simulink model "s0809"  (Simulink 6.0)
settings: Solver=ode45  SolverMode=SingleTasking  StartTime=0.0  StopTime=300  MaxStep=200  RelTol=1e-3  AbsTol=1e-6
values from neighbouring files (symbols this model uses):
  T = 1    [m0304.m]
settings Model: LastModifiedBy=Froriep
settings DataIOCC: LimitDataPoints=off  SaveOutput=off  TimeSaveName=t
settings OptimizationCC: BooleanDataType=off
settings DebuggingCC: SolverPrmCheckMsg=none
settings HardwareCC: TargetUnknown=on
settings STFCustomTargetCC: TargetFcnLib=ansi_tfl_tmw.mat  GenFloatMathFcnCalls=ANSI_C  ModelReferenceCompliant=off  SystemTargetFile=grt.tlc

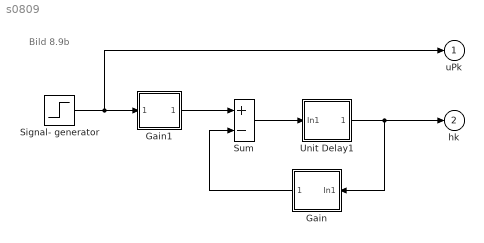
== system s0809 ==
  note: Bild 8.9b
  Gain : Subsystem  Orientation=left  mask{@1=a1}
      mask prompts: @1 "a1"
      mask help: Konstante
      mask init:
      | a1=@1;
      mask Display: disp('a1')
  Gain1 : Subsystem  mask{@1=b1}
      mask prompts: @1 "b0"
      mask help: Konstante
      mask init:
      | b1=@1;
      mask Display: disp('b1')
  Signal- generator : Step  Time=0  SampleTime=T
  Sum : Sum  Inputs=+-  SaturateOnIntegerOverflow=on  InputSameDT=on
  Unit Delay1 : Subsystem  mask{@1=T}
      mask prompts: @1 "T"
      mask help: Verschiebeglied
      mask init:
      | T=@1;
      mask Display: disp('T')
  uPk : Outport
  hk : Outport  Port=2
  wires:
  Signal- generator/1 -> uPk/1, Gain1/1(In1)
  Sum/1 -> Unit Delay1/1(In1)
  Gain1/1(Out1) -> Sum/1
  Gain/1(Out1) -> Sum/2
  Unit Delay1/1(Out1) -> Gain/1(In1), hk/1

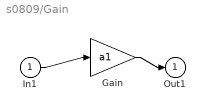
== system s0809/Gain ==
  In1 : Inport  Port=1  LatchInput=off
  Gain : Gain  Gain=a1  SaturateOnIntegerOverflow=on
  Out1 : Outport
  wires:
  In1/1 -> Gain/1
  Gain/1 -> Out1/1

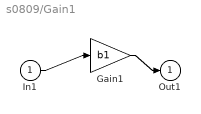
== system s0809/Gain1 ==
  In1 : Inport  Port=1  LatchInput=off
  Gain1 : Gain  Gain=b1  SaturateOnIntegerOverflow=on
  Out1 : Outport
  wires:
  In1/1 -> Gain1/1
  Gain1/1 -> Out1/1

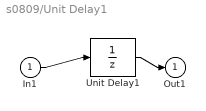
== system s0809/Unit Delay1 ==
  In1 : Inport  Port=1  LatchInput=off
  Unit Delay1 : UnitDelay  SampleTime=T
  Out1 : Outport
  wires:
  In1/1 -> Unit Delay1/1
  Unit Delay1/1 -> Out1/1
